simulink model "RotaryInvertedPendulumHardwareInLoop"  (R2020a)
settings: Solver=FixedStepAuto  StartTime=0.0  StopTime=inf  RelTol=1e-3  EnableMultiTasking=on
undefined symbols (not defined in the file or in its folder): k
libraries: arduinolib x3, simulink_extras x2, eeGeneralControl x2
settings Model: SILPILModeSetting=veronly  ExtModeTrigDuration=1  Creator=hima_  LastModifiedBy=hima_
settings OptimizationCC: EnhancedBackFolding=on  PassReuseOutputArgsAs=Individual arguments  ZeroExternalMemoryAtStartup=off  ZeroInternalMemoryAtStartup=off  MaxStackSize=64  OptimizeBlockOrder=speed  DifferentSizesBufferReuse=on  OptimizationCustomize=off  EfficientTunableParamExpr=on
settings DebuggingCC: ParameterTunabilityLossMsg=error
settings HardwareCC: ProdBitPerInt=16  ProdBitPerPointer=16  ProdBitPerSizeT=16  ProdBitPerPtrDiffT=16  ProdLargestAtomicFloat=None  ProdWordSize=8  ProdHWDeviceType=Atmel->AVR
settings SFSimCC: MATLABDynamicMemAlloc=off
settings RTWCC: SystemTargetFile=ert.tlc  HardwareBoard=Arduino Uno  TLCOptions=-aInlineSetEventsForThisBaseRateFcn=TLC_FALSE -aSuppressMultiTaskScheduler=TLC_FALSE -aRateBasedStepFcn=1  TemplateMakefile=ert_default_tmf  Toolchain=Arduino AVR  BuildConfiguration=Faster Runs
settings CodeAppCC: ForceParamTrailComments=on  IgnoreCustomStorageClasses=off  OperatorAnnotations=on  SimulinkDataObjDesc=on  SFDataObjDesc=on  InsertBlockDesc=on
settings ERTTargetCC: SupportContinuousTime=on  SupportVariableSizeSignals=on  ExtModeStaticAllocSize=250

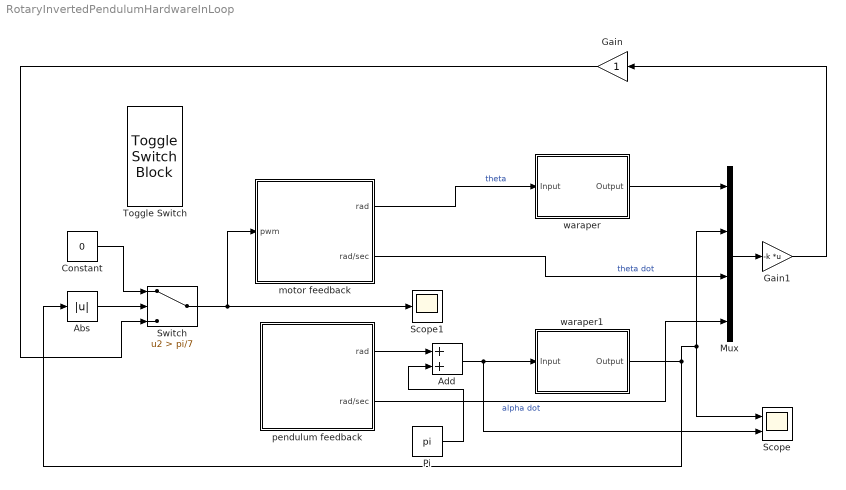
== system RotaryInvertedPendulumHardwareInLoop ==
  Abs : Abs
  Add : Sum
  Constant : Constant  Value=0
  Gain : Gain
  Gain1 : Gain  Gain=-k  Multiplication=Matrix(K*u)
  Mux : Mux
  Pi : Constant  Value=pi  OutDataTypeStr=Inherit: Inherit via back propagation
  Scope : Scope  NumInputPorts=2
  Scope1 : Scope
  Switch : Switch  Criteria=u2 > Threshold  Threshold=pi/7
  Toggle Switch : ToggleSwitchBlock
      settings: Values={{'Off', 'On'}, [0 1]}
  motor feedback : Subsystem
      mask Display: image('$imagefile'); % Use "Edit Image" on toolstrip to change.
  pendulum feedback : Subsystem
      mask Display: image('$imagefile'); % Use "Edit Image" on toolstrip to change.
  waraper : Subsystem
  waraper1 : Subsystem
  wires:
  Gain1/1 -> Gain/1
  motor feedback/2(rad/sec) -> Mux/3  "theta dot"
  pendulum feedback/2(rad/sec) -> Mux/4  "alpha dot"
  Mux/1 -> Gain1/1
  motor feedback/1(rad) -> waraper/1(Input)  "theta"
  waraper/1(Output) -> Mux/1
  waraper1/1(Output) -> Scope/1, Mux/2, Abs/1
  Add/1 -> Scope/2, waraper1/1(Input)
  Pi/1 -> Add/2
  Abs/1 -> Switch/2
  pendulum feedback/1(rad) -> Add/1
  Constant/1 -> Switch/1
  Switch/1 -> Scope1/1, motor feedback/1(pwm)
  Gain/1 -> Switch/3

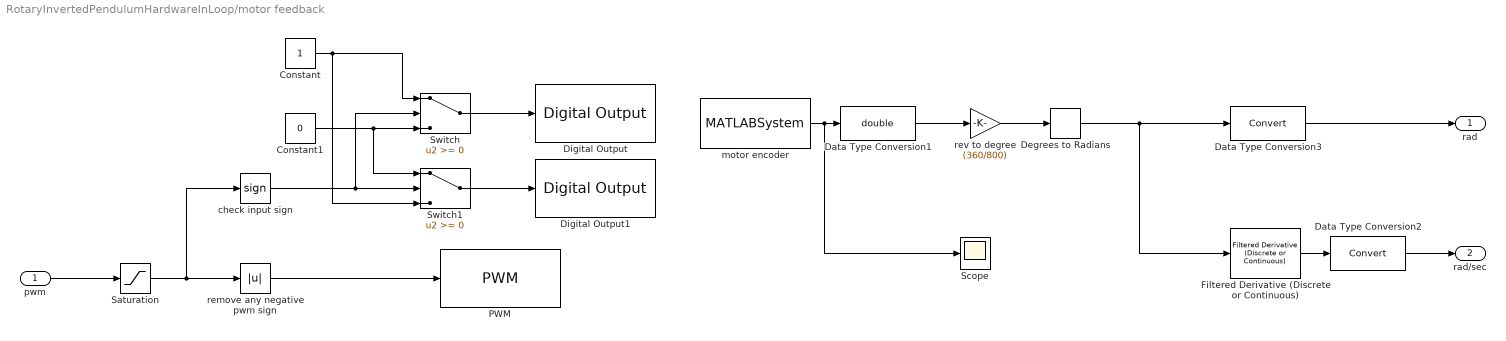
== system RotaryInvertedPendulumHardwareInLoop/motor feedback ==
  pwm : Inport
  Constant : Constant
  Constant1 : Constant  Value=0
  Data Type Conversion1 : DataTypeConversion  OutDataTypeStr=double
  Data Type Conversion2 : DataTypeConversion
  Data Type Conversion3 : DataTypeConversion
  Degrees to Radians : simulink_extras/Transformations/Degrees to Radians
  Digital Output : arduinolib/Digital Output  pinNumber=9  Direction=output  blockPlatform=arduino
  Digital Output1 : arduinolib/Digital Output  pinNumber=8  Direction=output  blockPlatform=arduino
  Filtered Derivative (Discrete or Continuous) : eeGeneralControl/Filtered Derivative (Discrete or Continuous)  K=-1  T=0.001  B=inf  A=-inf  minRatio=10  init_option=Inherited from block input  x0=0  Ts=-1
      settings: SourceProductBaseCode=PS
  PWM : arduinolib/PWM  pinNumber=6  frequencyType=Default  desiredFrequency=490.2  achievableFrequency=490.2
  Saturation : Saturate  UpperLimit=255  LowerLimit=-255
  Scope : Scope
  Switch : Switch
  Switch1 : Switch
  check input sign : Signum
  motor encoder : MATLABSystem  System=Encoder_arduino  Encoder=1  PinA=3  PinB=5  SampleTime=0.001
      mask Type: Encoder_arduino
      mask Display:
      | disp('Encoder');
      | port_label('output',1,'y');
  remove any negative pwm sign : Abs
  rev to degree : Gain  Gain=(360/800)
  rad : Outport
  rad/sec : Outport  Port=2
  wires:
  remove any negative pwm sign/1 -> PWM/1
  Saturation/1 -> check input sign/1, remove any negative pwm sign/1
  check input sign/1 -> Switch/2, Switch1/2
  Constant/1 -> Switch/1, Switch1/3
  Constant1/1 -> Switch1/1, Switch/3
  Switch/1 -> Digital Output/1
  Switch1/1 -> Digital Output1/1
  pwm/1 -> Saturation/1
  motor encoder/1 -> Scope/1, Data Type Conversion1/1
  Data Type Conversion1/1 -> rev to degree/1
  Data Type Conversion2/1 -> rad/sec/1
  Data Type Conversion3/1 -> rad/1
  rev to degree/1 -> Degrees to Radians/1
  Degrees to Radians/1 -> Filtered Derivative (Discrete or Continuous)/1, Data Type Conversion3/1
  Filtered Derivative (Discrete or Continuous)/1 -> Data Type Conversion2/1

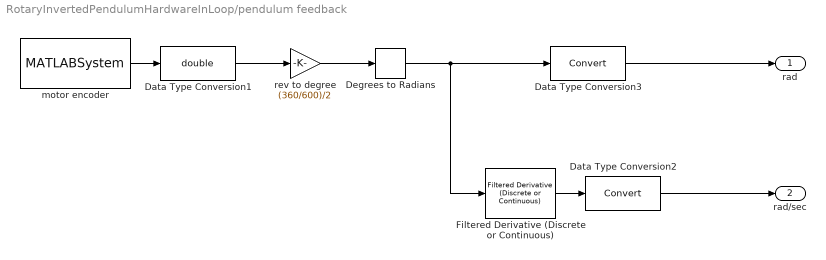
== system RotaryInvertedPendulumHardwareInLoop/pendulum feedback ==
  Data Type Conversion1 : DataTypeConversion  OutDataTypeStr=double
  Data Type Conversion2 : DataTypeConversion
  Data Type Conversion3 : DataTypeConversion
  Degrees to Radians : simulink_extras/Transformations/Degrees to Radians
  Filtered Derivative (Discrete or Continuous) : eeGeneralControl/Filtered Derivative (Discrete or Continuous)  K=1  T=0.001  B=inf  A=-inf  minRatio=10  init_option=Inherited from block input  x0=0  Ts=-1
      settings: SourceProductBaseCode=PS
  motor encoder : MATLABSystem  System=Encoder_arduino  Encoder=0  PinA=2  PinB=4  SampleTime=0.001
      mask Type: Encoder_arduino
      mask Display:
      | disp('Encoder');
      | port_label('output',1,'y');
  rev to degree : Gain  Gain=(360/600)/2
  rad : Outport
  rad/sec : Outport  Port=2
  wires:
  motor encoder/1 -> Data Type Conversion1/1
  Data Type Conversion3/1 -> rad/1
  Data Type Conversion2/1 -> rad/sec/1
  Data Type Conversion1/1 -> rev to degree/1
  rev to degree/1 -> Degrees to Radians/1
  Degrees to Radians/1 -> Filtered Derivative (Discrete or Continuous)/1, Data Type Conversion3/1
  Filtered Derivative (Discrete or Continuous)/1 -> Data Type Conversion2/1

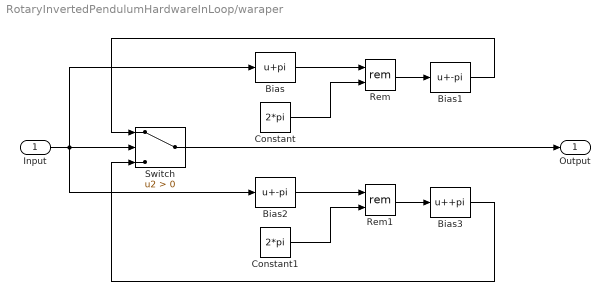
== system RotaryInvertedPendulumHardwareInLoop/waraper ==
  Input : Inport
  Bias : Bias  Bias=pi
  Bias1 : Bias  Bias=-pi
  Bias2 : Bias  Bias=-pi
  Bias3 : Bias  Bias=+pi
  Constant : Constant  Value=2*pi
  Constant1 : Constant  Value=2*pi
  Rem : Math  Operator=rem  SaturateOnIntegerOverflow=on
  Rem1 : Math  Operator=rem  SaturateOnIntegerOverflow=on
  Switch : Switch  Criteria=u2 > Threshold
  Output : Outport
  wires:
  Constant/1 -> Rem/2
  Bias/1 -> Rem/1
  Input/1 -> Bias/1, Bias2/1, Switch/2
  Bias3/1 -> Switch/3
  Bias2/1 -> Rem1/1
  Rem1/1 -> Bias3/1
  Constant1/1 -> Rem1/2
  Switch/1 -> Output/1
  Rem/1 -> Bias1/1
  Bias1/1 -> Switch/1

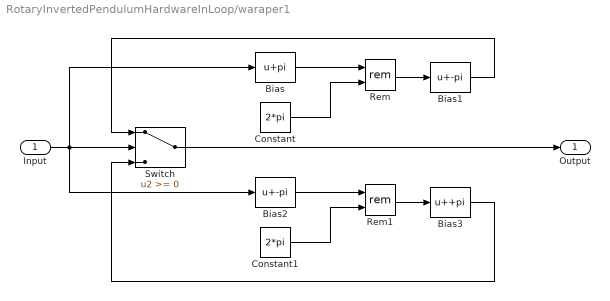
== system RotaryInvertedPendulumHardwareInLoop/waraper1 ==
  Input : Inport
  Bias : Bias  Bias=pi
  Bias1 : Bias  Bias=-pi
  Bias2 : Bias  Bias=-pi
  Bias3 : Bias  Bias=+pi
  Constant : Constant  Value=2*pi
  Constant1 : Constant  Value=2*pi
  Rem : Math  Operator=rem  SaturateOnIntegerOverflow=on
  Rem1 : Math  Operator=rem  SaturateOnIntegerOverflow=on
  Switch : Switch
  Output : Outport
  wires:
  Constant/1 -> Rem/2
  Bias/1 -> Rem/1
  Input/1 -> Bias/1, Bias2/1, Switch/2
  Bias3/1 -> Switch/3
  Bias2/1 -> Rem1/1
  Rem1/1 -> Bias3/1
  Constant1/1 -> Rem1/2
  Switch/1 -> Output/1
  Rem/1 -> Bias1/1
  Bias1/1 -> Switch/1
